simulink model "AM5_2"  (R2020b)
settings: Solver=VariableStepDiscrete  StartTime=0.0  StopTime=2  MaxStep=1/800  RelTol=1e-3
settings Model: Creator=seojoon  LastModifiedBy=seojoon

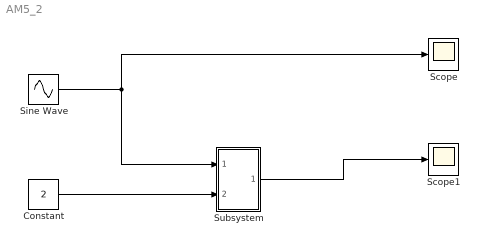
== system AM5_2 ==
  Constant : Constant  Value=2
  Scope : Scope
  Scope1 : Scope
  Sine Wave : Sin  Amplitude=2  Frequency=2*pi*5  SampleTime=0
  Subsystem : Subsystem
  wires:
  Sine Wave/1 -> Subsystem/1(In1), Scope/1
  Constant/1 -> Subsystem/2(In2)
  Subsystem/1(Out1) -> Scope1/1

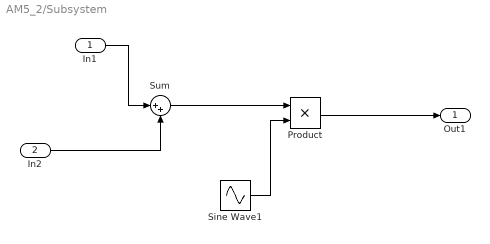
== system AM5_2/Subsystem ==
  In1 : Inport
  In2 : Inport  Port=2
  Product : Product
  Sine Wave1 : Sin  Frequency=2*pi*50  Phase=pi/2  SampleTime=0
  Sum : Sum  Inputs=|++
  Out1 : Outport
  wires:
  Sine Wave1/1 -> Product/2
  In2/1 -> Sum/2
  Sum/1 -> Product/1
  Product/1 -> Out1/1
  In1/1 -> Sum/1
